simulink model "delayed_integral_action"  (R2018b)
settings: Solver=VariableStepAuto  StartTime=0.0  StopTime=100.0  RelTol=1e-3
values from neighbouring files (symbols this model uses):
  dc_gain = dcgain(feedback_sys_discrete)    [control_input_bound.m]    (also in delayed_input.m; discrete_pole_placement.m)
  K = 20    [continous_controller.m]    (also in control_input_bound.m = place(sys_discrete.A, sys_discrete.B, discrete_poles); delayed_input.m = place(sys_discrete.A, sys_discrete.B, discrete_poles); discrete_pole_placement.m = place(sys_discrete.A, sys_discrete.B, discrete_poles); pole_placement_delay.m = place(sys.A, sys.B, continous_poles))
  sys_discrete = c2d(sys, 2*pi/sampling_freq, 'zoh')    [control_input_bound.m]    (also in delayed_input.m = (c2d(sys, 2*pi/sampling_freq, 'zoh')); discrete_pole_placement.m = (c2d(sys, 2*pi/sampling_freq, 'zoh')); discretization.m; lqr_controller.m)
undefined symbols (not defined in the file or in its folder): DiscIntNeverNeededParam
settings Model: Creator=lorenzoterenzi  LastModifiedBy=lorenzoterenzi

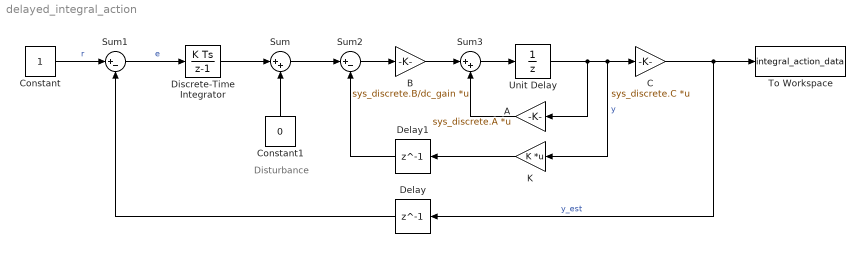
== system delayed_integral_action ==
  note: Disturbance
  A : Gain  Gain=sys_discrete.A  Multiplication=Matrix(K*u)
  B : Gain  Gain=sys_discrete.B/dc_gain  Multiplication=Matrix(K*u)
  C : Gain  Gain=sys_discrete.C  Multiplication=Matrix(K*u)
  Constant : Constant
  Constant1 : Constant  Value=0
  Delay : Delay  DelayLength=1
  Delay1 : Delay  DelayLength=1
  Discrete-Time Integrator : DiscreteIntegrator  gainval=0.5  SampleTime=-1  ICPrevOutput=DiscIntNeverNeededParam  ICPrevScaledInput=DiscIntNeverNeededParam
  K : Gain  Gain=K  Multiplication=Matrix(K*u)
  Sum : Sum  Inputs=|++
  Sum1 : Sum  Inputs=|+-
  Sum2 : Sum  Inputs=|+-
  Sum3 : Sum  Inputs=|++
  To Workspace : ToWorkspace  VariableName=integral_action_data  SaveFormat=Timeseries  SampleTime=-1
  Unit Delay : UnitDelay  SampleTime=sys_discrete.Ts
  wires:
  Constant/1 -> Sum1/1  "r"
  Discrete-Time Integrator/1 -> Sum/1
  Sum1/1 -> Discrete-Time Integrator/1  "e"
  Sum/1 -> Sum2/1
  Constant1/1 -> Sum/2
  K/1 -> Delay1/1
  Sum2/1 -> B/1
  Unit Delay/1 -> A/1, K/1, C/1  "y"
  A/1 -> Sum3/2
  B/1 -> Sum3/1
  Sum3/1 -> Unit Delay/1
  C/1 -> Delay/1, To Workspace/1  "y_est"
  Delay/1 -> Sum1/2
  Delay1/1 -> Sum2/2
